simulink model "SimulinkKalman"  (R2016a)
settings: Solver=FixedStepAuto  StartTime=0.0  StopTime=10.0  FixedStep=0.1  RelTol=1e-3
settings Model: Creator=김태욱  LastModifiedBy=김태욱

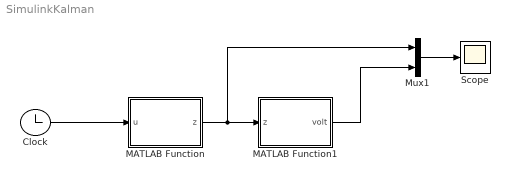
== system SimulinkKalman ==
  Clock : Clock
  MATLAB Function : MATLAB Function  TreatAsAtomicUnit=on
  MATLAB Function1 : MATLAB Function  TreatAsAtomicUnit=on
  Mux1 : Mux  Inputs=2
  Scope : Scope
  wires:
  Clock/1 -> MATLAB Function/1(u)
  Mux1/1 -> Scope/1
  MATLAB Function/1(z) -> Mux1/1, MATLAB Function1/1(z)
  MATLAB Function1/1(volt) -> Mux1/2

== matlab function SimulinkKalman/MATLAB Function1 ==
  data: z input; volt output
function volt = SimKalman(z)
%#codegen
% persistent vriables : only in function variables
% for initialization it is good
% 
persistent Phi H G V            
persistent xEst P
persistent firstRun


if isempty(firstRun)     % at first firstREun = 0                              
  Phi = 1;
  H = 1;  
  G = 0;
  V =2;
  xEst = 14;
  P =  4;  
  firstRun = 1;  
end  
xPre = Phi*xEst;
M = Phi*P*Phi' + G;
K = M*H'*inv(H*M*H' + V);
xEst = xPre + K*(z - H*xPre);
P = M - K*H*M;
volt = xEst;
% Cov = P;

== matlab function SimulinkKalman/MATLAB Function ==
  data: u input; z output
function z = SimMeas(u)
%#codegen
w = 0 + 4*randn(1,1);    %  zero mean and variance = 4*4 
z = 10 + w;                 %  measurement
